simulink model "Copter_Plane_h2g_4_and_1_20200824"  (R2020a)
settings: Solver=ode1  StartTime=0.0  StopTime=100  FixedStep=dt  RelTol=1e-3
values from neighbouring files (symbols this model uses):
  HD = 180/pi    (= 57.2957795131)    [mode_data.m]
undefined symbols (not defined in the file or in its folder): center_WP, GRAVITY_MSS, gyro_x, gyro_y, gyro_z, J, Kd, Ku, Ld, Ldx, Ldy, Lu, Lux, Luy, m_kg, Newton, pitch, pwm_max, pwm_min, Qd, QLd, QLdx, QLdy, QLu, QLux, QLuy, Qu, Raphson, roll, vel_desired, yaw
libraries: shared6dofsys x3, sharedutil x1, simulink x1, aerolibasang x1
(part 2 of 2)

== matlab function Copter_Plane_h2g_4_and_1_20200824/pland_mode/pland_F_M_4a1 ==
  settings: updateMethod=DISCRETE
  data: F output; k_rudder input; k_aileron input; k_throttle input; k_elevator input; wx input; wy input; wz input; alpha input; beta input; V input; alt input; M output; mode input; pwm_out input; Ku parameter; Kd parameter; Lux parameter; Luy parameter; Ldx parameter; Ldy parameter; Lu parameter; Ld parameter; pwm_min parameter; pwm_max parameter; Qu parameter; Qd parameter; tail_tilt data_store_memory; QLux parameter; QLuy parameter; QLu parameter; QLdx parameter; QLdy parameter; QLd parameter; pwm_tail data_store_memory
function [F,M]   = pland_F_M_4a1(k_rudder,k_aileron,k_throttle,k_elevator,wx,wy,wz,alpha,beta,V,alt,mode,pwm_out, Ku, Kd, Lux, Luy, Ldx, Ldy, Lu, Ld, pwm_min, pwm_max, Qu, Qd, QLux, QLuy, QLu, QLdx, QLdy, QLd)
    
%鎺ㄥ姏妯″瀷锛孴hr=throttle_dem*Tmax锛宼hrottle_dem=24N銆俓n%闃诲姏妯″瀷锛孋x_Sref=Cx_Sref_alpha*alpha,Cx_Sref_alpha=0.007;
%鍗囧姏妯″瀷  Cy_Sref=Cy_Sref_alpha*(alpha0+alpha),Cy_Sref_alpha=0.022,alpha0=5;
%%%%%%%%%%%%%%%%%%%%%%%%%%%%%%%%%%%%%%%%%%%%%%%%%%%%%%%%%%%%%%%%%%%%%%%
global tail_tilt
global pwm_tail
Tmax=26*9.8*0.6;
HD=180/pi;
% if(abs(alpha)>20/HD||V<8)
%     V=0;
% end
if(V<8)
    V=0;
end

alpha=constrain_value(alpha,-10/HD,10/HD);
beta=constrain_value(beta,-10/HD,10/HD);
Cx_Sref_alpha=-1.274/2/10;%8/144.5
Cz_Sref_alpha=-1.274/2;
Cy_Sref_beta=-1.274/2/10;
alpha0=2/HD;
Cx_Sref=Cx_Sref_alpha*20;
Cy_Sref=Cy_Sref_beta*(beta)*HD;
Cz_Sref=Cz_Sref_alpha*(alpha+alpha0)*HD;

Sbw=[cos(alpha)*cos(beta)   -cos(alpha)*sin(beta)   -sin(alpha)
    sin(beta)               cos(beta)               0
    sin(alpha)*cos(beta)    -sin(alpha)*sin(beta)   cos(alpha)];
[~,~,rho,~] = atom_mode(alt+2000);
q=0.5*rho*V*V;
D=q*Cx_Sref;%+k_throttle*Tmax;
C=q*Cy_Sref;
L=q*Cz_Sref;
Fw=[D; C; L];
Fb=Sbw*Fw;
TF=(pwm_tail-pwm_min)/(pwm_max-pwm_min)*Tmax;
F_Plane=Fb+[TF;0;0];
% F_Plane=Fb;

%%%%%%%%%%%%%%%%%%%%%%%%%%%%%%%%%%%%%%%%%%%%%%%%%
dl=0.1;
Mby=Fb(3)*dl;
Mbz=-Fb(2)*dl;
%%%%%%%%%%%%%%%%%%%%%%%%%
dmxa=71.8362;    %(2*pi*5)^2*Jx/HD
dmx_wx=0.1;
%%%%%%%%%%%%%%%%%%%%%%%%%%%
dmya=q*Cz_Sref_alpha*dl;  %(2*pi*1.5)^2*Jy/HD
dmye=-dmya/2;
dmy_wy=0.2;
%%%%%%%%%%%%%%%%%%%%%%%%%
dmzb=-q*Cy_Sref_beta*dl;    %(2*pi*5)^2*Jx/HD
dmzr=dmzb*0.3;
dmz_wz=0.2;
%%%%%%%%%%%%%%%%%%%%%%%%
Mx=dmxa*k_aileron/100          -dmx_wx*wx;
My=dmye*(k_elevator+680)/100  +Mby   -dmy_wy*wy;
% My=dmye*(k_elevator)/100  +Mby   -dmy_wy*wy;
Mz=dmzr*k_rudder/100    +Mbz   -dmz_wz*wz;
M_Plane=[Mx; My ;Mz];
%%%%%%%%%%%%%%%%%%%%%%%%%%%%%%%%%%%%%%%%%%%%%%%%%%%%%%%%%%%%%%%%%%%
%%%%%%%%%%%%%%%%%%%%%%%%%%%%%%%%%%%%%%%%%%%%%%%%%%%%%%%%%%%%%%%%%%%%%
%%%%%%%%%%%%%%%%%%%%%%%%%%%%%%%%%%%%%%%%%%%%%%%%%%%%%%%%%%%%%%%%%%%%%
Ku_v10=26*9.8*3/4;
F1=(pwm_out(1)-pwm_min)/(pwm_max-pwm_min)*Ku_v10;
F2=(pwm_out(2)-pwm_min)/(pwm_max-pwm_min)*Ku_v10;
F3=(pwm_out(3)-pwm_min)/(pwm_max-pwm_min)*Ku_v10;
F4=(pwm_out(4)-pwm_min)/(pwm_max-pwm_min)*Ku_v10;

tail_tilt_temp=constrain_value(tail_tilt,-9000,700);

F24x_g=(F2+F4)*sind(-tail_tilt_temp/100);
F24z_g=(F2+F4)*cosd(-tail_tilt_temp/100);

F_copter=[F24x_g; 0 ;-(F1+F3+F24z_g)];
L_v10=0.5;
Q=4.5;
Mx=(-F1+F3)*L_v10+(F2-F4)*L_v10;
% My=(F1+F3)*Luy+(-F2-F4)*Ldy;
My=(F1+F3)*L_v10+(-F2-F4)*L_v10*cosd(-tail_tilt_temp/100);
Mz=(-F1+F3)*L_v10*sind(Q)+(-F2+F4)*L_v10*sind(Q);%0.1736=sind(10)  0.1071= Ld*900*sind(10)/(Lu*1600)
Mz_g=(F2-F4)*Ldx*sind(-tail_tilt_temp/100);
% Mz_g=0;
Mz=Mz+Mz_g;
M_copter=[Mx; My; Mz];
%%%%%%%%%%%%%%%%%%%%%%%%%%%%%%%%%%%%%%%%%%%%%%%%%%%%%%%
%% 0 :copter Stabilize,1:copter althold ,2:copter poshold,3:Plane Stabilize 4:Plane TECS; 5：Plane L1
    F=F_copter+F_Plane;
    M=M_copter+M_Plane;
    
%     F=F_copter;
%     M=M_copter;
%%%%%%%%%%%%%%%%%%%%%%%%%%%%%%%%%%%%%%%%%%%%%%%%%%%%%%%%%%%%
end
